simulink model "CryoDetHcd"  (R2016b)
settings: Solver=ode45  StartTime=0.0  StopTime=1e-3  RelTol=1e-3
PreLoadFcn:
  | setup_hcd
values from neighbouring files (symbols this model uses):
  A = sqrt(0.5*erfc(x))    [setup_hcd.m]
  Fadc = 307.2e6    (= 307200000)    [setupADCtoDACloopback.m]    (also in setupCryoFPGA_CMB.m; setup_hcd.m = 614000000)
undefined symbols (not defined in the file or in its folder): AXI4, B, C, D, etaRomData, freqRomData, freqRomData1, freqRomData2, freqRomData3, j, Lite
libraries: xbsIndex_r4 x897, CryoDetLibCMB x8, hdlsllib x8, dspsigops x2, simulink x1
(part 8 of 8)

== system CryoDetHcd/DspCore/DSP/channel_processor/channel_processor_x4/freqWord_debug/alpha_filter1 ==
  In1 : Inport
  alpha : Inport  Port=2
  ch : Inport  Port=3
  (D-A)*B + C : xbsIndex_r4/DSP48 Macro 3.0   dsptype=Target XtremeDSP Slice: DSP48E2  instruction_list=(D-A)*B+C  AvailableInstructions=|  show_filtered=on  pipeline_options=Expert  dspimage=?  tier_1=off  tier_2=off  tier_3=off  tier_4=off  tier_5=off  tier_6=off  dreg_1=off  dreg_2=off  dreg_3=on  areg_1=off  areg_2=off  areg_3=on  areg_4=on  breg_1=off  breg_2=off  breg_3=on  breg_4=on  mreg_5=on  concatreg_3=off  concatreg_4=off  concatreg_5=off  creg_1=off  creg_2=off  creg_3=on  creg_4=on  creg_5=on  preg_6=on  cinreg_1=off  cinreg_2=off  cinreg_3=off  cinreg_4=off  cinreg_5=off  opreg_1=off  opreg_2=off  opreg_3=off  opreg_4=off  opreg_5=off  output_properties=Full_Precision  p_width=48  p_binarywidth=0  has_acout=off  has_bcout=off  has_pcout=off  has_carryout=off  has_carrycascout=off  has_ce=off  has_d_ce=off  has_a_ce=off  has_b_ce=off  has_concat_ce=off  has_c_ce=off  has_m_ce=off  has_p_ce=off  has_sel_ce=off  has_sclr=off  has_d_sclr=off  has_a_sclr=off  has_b_sclr=off  has_concat_sclr=off  has_c_sclr=off  has_m_sclr=off  has_p_sclr=off  has_sel_sclr=off  use_dsp48=on  simulation_type=fast_sim  simulation_model=sysgen:xbip_dsp48_macro_v3_0  gui_behaviour=Sysgen  instruction1='#'  ip_name=DSP48 Macro  ip_version=3.0  dsptool_ready=true  ipcore_usecache=true  ipcore_useipmodelcache=true  wrapper_available=true  port_translation_map={ 'ce' => 'en', 'sclr' => 'rst'}  ipcore_latency_function='has_combinational'  structural_sim=false  ipcore_verbose=false  ipcore_port_config={ 'carryin' => { 'arith' => 'ufix', 'binpt' => 0.00000000000, 'width' => 1.00000000000}, 'carrycascin' => { 'arith' => 'ufix', 'binpt' => 0.00000000000, 'width' => 1.00000000000}, 'carrycascout' => { 'arith' => 'ufix', 'binpt' => 0.00000000000, 'width' => 1.00000000000}, 'carryout' => { 'arith' => 'ufix', 'binpt' => 0.00000000000, 'width' => 1.00000000000}}  ipcore_xco_need_fpga_part=true  block_type=xbip_dsp48_macro_v3_0
      | (D-A)*B+C
      | (D-A)*B+C+C
      | (D-A)*B+C+C+CARRYIN
      | (D-A)*B+C+CARRYIN
      | (D-A)*B+C+P
      | (D-A)*B+C+P+CARRYIN
      | (D-A)*B+C+P>>17
      | (D-A)*B+C+P>>17+CARRYIN
      | (D-A)*B+C+PCIN
      | (D-A)*B+C+PCIN+CARRYIN
      | (D-A)*B+C+PCIN>>17
      | (D-A)*B+C+PCIN>>17+CARRYIN
      | (D-A)*B+C-C
      | (D-A)*B+C-P
      | (D-A)*B+C-P>>17
      | (D-A)*B+C-PCIN
      | (D-A)*B+C-PCIN>>17
      | (D-A)*B+CARRYIN
      | -((D-A)*B+C)
      | -((D-A)*B+C+CARRYIN)
      | -((D-A)*B+CARRYIN)
      | -(C+(D-A)*B+CARRYIN)
      | -(P+(D-A)*B+CARRYIN)
      | -C+(D-A)*B+C
      | -P+(D-A)*B+C
      | -P>>17+(D-A)*B+C
      | -PCIN+(D-A)*B+C
      | -PCIN>>17+(D-A)*B+C
      | C+(D-A)*B+C
      | C+(D-A)*B+C+CARRYIN
      | C+(D-A)*B+CARRYIN
      | C+C+(D-A)*B+CARRYIN
      | C+P+(D-A)*B+CARRYIN
      | C+P>>17+(D-A)*B+CARRYIN
      | C+PCIN+(D-A)*B+CARRYIN
      | C+PCIN>>17+(D-A)*B+CARRYIN
      | C-((D-A)*B+C)
      | C-((D-A)*B+C+CARRYIN)
      | C-((D-A)*B+CARRYIN)
      | C-(C+(D-A)*B+CARRYIN)
      | C-(P+(D-A)*B+CARRYIN)
      | P+(D-A)*B+C
      | P+(D-A)*B+C+CARRYIN
      | P+(D-A)*B+CARRYIN
      | P+C+(D-A)*B+CARRYIN
      | P+P+(D-A)*B+CARRYIN
      | P+P>>17+(D-A)*B+CARRYIN
      | P+PCIN+(D-A)*B+CARRYIN
      | P+PCIN>>17+(D-A)*B+CARRYIN
      | P-((D-A)*B+C)
      | P-((D-A)*B+C+CARRYIN)
      | P-((D-A)*B+CARRYIN)
      | P-(C+(D-A)*B+CARRYIN)
      | P-(P+(D-A)*B+CARRYIN)
      | P>>17+(D-A)*B+C
      | P>>17+(D-A)*B+C+CARRYIN
      | P>>17+(D-A)*B+CARRYIN
      | P>>17+C+(D-A)*B+CARRYIN
      | P>>17+P+(D-A)*B+CARRYIN
      | P>>17-((D-A)*B+C)
      | P>>17-((D-A)*B+C+CARRYIN)
      | P>>17-((D-A)*B+CARRYIN)
      | P>>17-(C+(D-A)*B+CARRYIN)
      | P>>17-(P+(D-A)*B+CARRYIN)
      | PCIN+(D-A)*B+C
      | PCIN+(D-A)*B+C+CARRYIN
      | PCIN+(D-A)*B+CARRYIN
      | PCIN+C+(D-A)*B+CARRYIN
      | PCIN+P+(D-A)*B+CARRYIN
      | PCIN-((D-A)*B+C)
      | PCIN-((D-A)*B+C+CARRYIN)
      | PCIN-((D-A)*B+CARRYIN)
      | PCIN-(C+(D-A)*B+CARRYIN)
      | PCIN-(P+(D-A)*B+CARRYIN)
      | PCIN>>17+(D-A)*B+C
      | PCIN>>17+(D-A)*B+C+CARRYIN
      | PCIN>>17+(D-A)*B+CARRYIN
      | PCIN>>17+C+(D-A)*B+CARRYIN
      | PCIN>>17+P+(D-A)*B+CARRYIN
      | PCIN>>17-((D-A)*B+C)
      | PCIN>>17-((D-A)*B+C+CARRYIN)
      | PCIN>>17-((D-A)*B+CARRYIN)
      | PCIN>>17-(C+(D-A)*B+CARRYIN)
      | PCIN>>17-(P+(D-A)*B+CARRYIN)
      | RNDMACC((D-A)*B+C+P)
      | RNDSIMPLE((D-A)*B+C)
      | RNDSIMPLE((D-A)*B+C+CARRYIN)
      | RNDSIMPLE((D-A)*B+CARRYIN)
      | RNDSIMPLE(C+(D-A)*B+CARRYIN)
      | RNDSIMPLE(P+(D-A)*B+CARRYIN)
      | RNDSIMPLE(P>>17+(D-A)*B+CARRYIN)
      | RNDSIMPLE(PCIN+(D-A)*B+CARRYIN)
      | RNDSIMPLE(PCIN>>17+(D-A)*B+CARRYIN)
      settings: infoedit=<html>Valid operands: CONCAT, P, C, PCIN, P>>17, PCIN>>17, CARRYIN, CARRYCASCIN, ACIN, A, BCIN,B<br><br>Valid operators: +, -, *, ()<br><br>Valid functions: RNDSIMPLE, RNDSYM<br><br>Instructions are case insensitive and tolerate spaces.</html>
  Convert : xbsIndex_r4/Convert  gui_display_data_type=Fixed-point  arith_type=Unsigned  n_bits=24  bin_pt=0  float_type=Single  exp_bits=8  fraction_bits=24  quantization=Truncate  overflow=Wrap  en=off  latency=0  pipeline=off  dbl_ovrd=off  block_type=convert
  Convert1 : xbsIndex_r4/Convert  gui_display_data_type=Fixed-point  arith_type="Signed  (2's comp)"  n_bits=25  bin_pt=0  float_type=Single  exp_bits=8  fraction_bits=24  quantization=Truncate  overflow=Wrap  en=off  latency=0  pipeline=off  dbl_ovrd=off  block_type=convert
  Convert2 : xbsIndex_r4/Convert  gui_display_data_type=Fixed-point  arith_type="Signed  (2's comp)"  n_bits=18  bin_pt=15  float_type=Single  exp_bits=8  fraction_bits=24  quantization=Truncate  overflow=Wrap  en=off  latency=0  pipeline=off  dbl_ovrd=off  block_type=convert
  Convert3 : xbsIndex_r4/Convert  gui_display_data_type=Fixed-point  arith_type="Signed  (2's comp)"  n_bits=25  bin_pt=0  float_type=Single  exp_bits=8  fraction_bits=24  quantization=Truncate  overflow=Wrap  en=off  latency=0  pipeline=off  dbl_ovrd=off  block_type=convert
  Delay : xbsIndex_r4/Delay  rst=off  infoeditControl=Selection of Reset will increase slice count due to use of real FFs and instead of SRLs  en=off  latency=124  reg_retiming=off  dbl_ovrd=off  block_type=delay
  Delay1 : xbsIndex_r4/Delay  rst=off  infoeditControl=Selection of Reset will increase slice count due to use of real FFs and instead of SRLs  en=off  latency=4  reg_retiming=off  dbl_ovrd=off  block_type=delay
  Register : xbsIndex_r4/Register  init=0  rst=off  en=off  dbl_ovrd=off  block_type=register
  Out1 : Outport
  ch_o : Outport  Port=2
  wires:
  alpha/1 -> Convert2/1
  Delay1/1 -> ch_o/1
  ch/1 -> Delay1/1
  Convert3/1 -> (D-A)*B + C/1
  Convert2/1 -> (D-A)*B + C/3
  Convert/1 -> Out1/1
  Convert1/1 -> (D-A)*B + C/2
  (D-A)*B + C/1 -> Delay/1, Convert/1
  Delay/1 -> (D-A)*B + C/4, Convert1/1
  In1/1 -> Register/1
  Register/1 -> Convert3/1

== system CryoDetHcd/DspCore/DSP/channel_processor/channel_processor_x4/freqWord_debug/alpha_filter2 ==
  In1 : Inport
  alpha : Inport  Port=2
  ch : Inport  Port=3
  (D-A)*B + C : xbsIndex_r4/DSP48 Macro 3.0   dsptype=Target XtremeDSP Slice: DSP48E2  instruction_list=(D-A)*B+C  AvailableInstructions=|  show_filtered=on  pipeline_options=Expert  dspimage=?  tier_1=off  tier_2=off  tier_3=off  tier_4=off  tier_5=off  tier_6=off  dreg_1=off  dreg_2=off  dreg_3=on  areg_1=off  areg_2=off  areg_3=on  areg_4=on  breg_1=off  breg_2=off  breg_3=on  breg_4=on  mreg_5=on  concatreg_3=off  concatreg_4=off  concatreg_5=off  creg_1=off  creg_2=off  creg_3=on  creg_4=on  creg_5=on  preg_6=on  cinreg_1=off  cinreg_2=off  cinreg_3=off  cinreg_4=off  cinreg_5=off  opreg_1=off  opreg_2=off  opreg_3=off  opreg_4=off  opreg_5=off  output_properties=Full_Precision  p_width=48  p_binarywidth=0  has_acout=off  has_bcout=off  has_pcout=off  has_carryout=off  has_carrycascout=off  has_ce=off  has_d_ce=off  has_a_ce=off  has_b_ce=off  has_concat_ce=off  has_c_ce=off  has_m_ce=off  has_p_ce=off  has_sel_ce=off  has_sclr=off  has_d_sclr=off  has_a_sclr=off  has_b_sclr=off  has_concat_sclr=off  has_c_sclr=off  has_m_sclr=off  has_p_sclr=off  has_sel_sclr=off  use_dsp48=on  simulation_type=fast_sim  simulation_model=sysgen:xbip_dsp48_macro_v3_0  gui_behaviour=Sysgen  instruction1='#'  ip_name=DSP48 Macro  ip_version=3.0  dsptool_ready=true  ipcore_usecache=true  ipcore_useipmodelcache=true  wrapper_available=true  port_translation_map={ 'ce' => 'en', 'sclr' => 'rst'}  ipcore_latency_function='has_combinational'  structural_sim=false  ipcore_verbose=false  ipcore_port_config={ 'carryin' => { 'arith' => 'ufix', 'binpt' => 0.00000000000, 'width' => 1.00000000000}, 'carrycascin' => { 'arith' => 'ufix', 'binpt' => 0.00000000000, 'width' => 1.00000000000}, 'carrycascout' => { 'arith' => 'ufix', 'binpt' => 0.00000000000, 'width' => 1.00000000000}, 'carryout' => { 'arith' => 'ufix', 'binpt' => 0.00000000000, 'width' => 1.00000000000}}  ipcore_xco_need_fpga_part=true  block_type=xbip_dsp48_macro_v3_0
      | (D-A)*B+C
      | (D-A)*B+C+C
      | (D-A)*B+C+C+CARRYIN
      | (D-A)*B+C+CARRYIN
      | (D-A)*B+C+P
      | (D-A)*B+C+P+CARRYIN
      | (D-A)*B+C+P>>17
      | (D-A)*B+C+P>>17+CARRYIN
      | (D-A)*B+C+PCIN
      | (D-A)*B+C+PCIN+CARRYIN
      | (D-A)*B+C+PCIN>>17
      | (D-A)*B+C+PCIN>>17+CARRYIN
      | (D-A)*B+C-C
      | (D-A)*B+C-P
      | (D-A)*B+C-P>>17
      | (D-A)*B+C-PCIN
      | (D-A)*B+C-PCIN>>17
      | (D-A)*B+CARRYIN
      | -((D-A)*B+C)
      | -((D-A)*B+C+CARRYIN)
      | -((D-A)*B+CARRYIN)
      | -(C+(D-A)*B+CARRYIN)
      | -(P+(D-A)*B+CARRYIN)
      | -C+(D-A)*B+C
      | -P+(D-A)*B+C
      | -P>>17+(D-A)*B+C
      | -PCIN+(D-A)*B+C
      | -PCIN>>17+(D-A)*B+C
      | C+(D-A)*B+C
      | C+(D-A)*B+C+CARRYIN
      | C+(D-A)*B+CARRYIN
      | C+C+(D-A)*B+CARRYIN
      | C+P+(D-A)*B+CARRYIN
      | C+P>>17+(D-A)*B+CARRYIN
      | C+PCIN+(D-A)*B+CARRYIN
      | C+PCIN>>17+(D-A)*B+CARRYIN
      | C-((D-A)*B+C)
      | C-((D-A)*B+C+CARRYIN)
      | C-((D-A)*B+CARRYIN)
      | C-(C+(D-A)*B+CARRYIN)
      | C-(P+(D-A)*B+CARRYIN)
      | P+(D-A)*B+C
      | P+(D-A)*B+C+CARRYIN
      | P+(D-A)*B+CARRYIN
      | P+C+(D-A)*B+CARRYIN
      | P+P+(D-A)*B+CARRYIN
      | P+P>>17+(D-A)*B+CARRYIN
      | P+PCIN+(D-A)*B+CARRYIN
      | P+PCIN>>17+(D-A)*B+CARRYIN
      | P-((D-A)*B+C)
      | P-((D-A)*B+C+CARRYIN)
      | P-((D-A)*B+CARRYIN)
      | P-(C+(D-A)*B+CARRYIN)
      | P-(P+(D-A)*B+CARRYIN)
      | P>>17+(D-A)*B+C
      | P>>17+(D-A)*B+C+CARRYIN
      | P>>17+(D-A)*B+CARRYIN
      | P>>17+C+(D-A)*B+CARRYIN
      | P>>17+P+(D-A)*B+CARRYIN
      | P>>17-((D-A)*B+C)
      | P>>17-((D-A)*B+C+CARRYIN)
      | P>>17-((D-A)*B+CARRYIN)
      | P>>17-(C+(D-A)*B+CARRYIN)
      | P>>17-(P+(D-A)*B+CARRYIN)
      | PCIN+(D-A)*B+C
      | PCIN+(D-A)*B+C+CARRYIN
      | PCIN+(D-A)*B+CARRYIN
      | PCIN+C+(D-A)*B+CARRYIN
      | PCIN+P+(D-A)*B+CARRYIN
      | PCIN-((D-A)*B+C)
      | PCIN-((D-A)*B+C+CARRYIN)
      | PCIN-((D-A)*B+CARRYIN)
      | PCIN-(C+(D-A)*B+CARRYIN)
      | PCIN-(P+(D-A)*B+CARRYIN)
      | PCIN>>17+(D-A)*B+C
      | PCIN>>17+(D-A)*B+C+CARRYIN
      | PCIN>>17+(D-A)*B+CARRYIN
      | PCIN>>17+C+(D-A)*B+CARRYIN
      | PCIN>>17+P+(D-A)*B+CARRYIN
      | PCIN>>17-((D-A)*B+C)
      | PCIN>>17-((D-A)*B+C+CARRYIN)
      | PCIN>>17-((D-A)*B+CARRYIN)
      | PCIN>>17-(C+(D-A)*B+CARRYIN)
      | PCIN>>17-(P+(D-A)*B+CARRYIN)
      | RNDMACC((D-A)*B+C+P)
      | RNDSIMPLE((D-A)*B+C)
      | RNDSIMPLE((D-A)*B+C+CARRYIN)
      | RNDSIMPLE((D-A)*B+CARRYIN)
      | RNDSIMPLE(C+(D-A)*B+CARRYIN)
      | RNDSIMPLE(P+(D-A)*B+CARRYIN)
      | RNDSIMPLE(P>>17+(D-A)*B+CARRYIN)
      | RNDSIMPLE(PCIN+(D-A)*B+CARRYIN)
      | RNDSIMPLE(PCIN>>17+(D-A)*B+CARRYIN)
      settings: infoedit=<html>Valid operands: CONCAT, P, C, PCIN, P>>17, PCIN>>17, CARRYIN, CARRYCASCIN, ACIN, A, BCIN,B<br><br>Valid operators: +, -, *, ()<br><br>Valid functions: RNDSIMPLE, RNDSYM<br><br>Instructions are case insensitive and tolerate spaces.</html>
  Convert : xbsIndex_r4/Convert  gui_display_data_type=Fixed-point  arith_type=Unsigned  n_bits=24  bin_pt=0  float_type=Single  exp_bits=8  fraction_bits=24  quantization=Truncate  overflow=Wrap  en=off  latency=0  pipeline=off  dbl_ovrd=off  block_type=convert
  Convert1 : xbsIndex_r4/Convert  gui_display_data_type=Fixed-point  arith_type="Signed  (2's comp)"  n_bits=25  bin_pt=0  float_type=Single  exp_bits=8  fraction_bits=24  quantization=Truncate  overflow=Wrap  en=off  latency=0  pipeline=off  dbl_ovrd=off  block_type=convert
  Convert2 : xbsIndex_r4/Convert  gui_display_data_type=Fixed-point  arith_type="Signed  (2's comp)"  n_bits=18  bin_pt=15  float_type=Single  exp_bits=8  fraction_bits=24  quantization=Truncate  overflow=Wrap  en=off  latency=0  pipeline=off  dbl_ovrd=off  block_type=convert
  Convert3 : xbsIndex_r4/Convert  gui_display_data_type=Fixed-point  arith_type="Signed  (2's comp)"  n_bits=25  bin_pt=0  float_type=Single  exp_bits=8  fraction_bits=24  quantization=Truncate  overflow=Wrap  en=off  latency=0  pipeline=off  dbl_ovrd=off  block_type=convert
  Delay : xbsIndex_r4/Delay  rst=off  infoeditControl=Selection of Reset will increase slice count due to use of real FFs and instead of SRLs  en=off  latency=124  reg_retiming=off  dbl_ovrd=off  block_type=delay
  Delay1 : xbsIndex_r4/Delay  rst=off  infoeditControl=Selection of Reset will increase slice count due to use of real FFs and instead of SRLs  en=off  latency=4  reg_retiming=off  dbl_ovrd=off  block_type=delay
  Register : xbsIndex_r4/Register  init=0  rst=off  en=off  dbl_ovrd=off  block_type=register
  Out1 : Outport
  ch_o : Outport  Port=2
  wires:
  alpha/1 -> Convert2/1
  Delay1/1 -> ch_o/1
  ch/1 -> Delay1/1
  Convert3/1 -> (D-A)*B + C/1
  Convert2/1 -> (D-A)*B + C/3
  Convert/1 -> Out1/1
  Convert1/1 -> (D-A)*B + C/2
  (D-A)*B + C/1 -> Delay/1, Convert/1
  Delay/1 -> (D-A)*B + C/4, Convert1/1
  In1/1 -> Register/1
  Register/1 -> Convert3/1

== system CryoDetHcd/DspCore/DSP/channel_processor/channel_processor_x4/freqWord_debug/alpha_filter3 ==
  In1 : Inport
  alpha : Inport  Port=2
  ch : Inport  Port=3
  (D-A)*B + C : xbsIndex_r4/DSP48 Macro 3.0   dsptype=Target XtremeDSP Slice: DSP48E2  instruction_list=(D-A)*B+C  AvailableInstructions=|  show_filtered=on  pipeline_options=Expert  dspimage=?  tier_1=off  tier_2=off  tier_3=off  tier_4=off  tier_5=off  tier_6=off  dreg_1=off  dreg_2=off  dreg_3=on  areg_1=off  areg_2=off  areg_3=on  areg_4=on  breg_1=off  breg_2=off  breg_3=on  breg_4=on  mreg_5=on  concatreg_3=off  concatreg_4=off  concatreg_5=off  creg_1=off  creg_2=off  creg_3=on  creg_4=on  creg_5=on  preg_6=on  cinreg_1=off  cinreg_2=off  cinreg_3=off  cinreg_4=off  cinreg_5=off  opreg_1=off  opreg_2=off  opreg_3=off  opreg_4=off  opreg_5=off  output_properties=Full_Precision  p_width=48  p_binarywidth=0  has_acout=off  has_bcout=off  has_pcout=off  has_carryout=off  has_carrycascout=off  has_ce=off  has_d_ce=off  has_a_ce=off  has_b_ce=off  has_concat_ce=off  has_c_ce=off  has_m_ce=off  has_p_ce=off  has_sel_ce=off  has_sclr=off  has_d_sclr=off  has_a_sclr=off  has_b_sclr=off  has_concat_sclr=off  has_c_sclr=off  has_m_sclr=off  has_p_sclr=off  has_sel_sclr=off  use_dsp48=on  simulation_type=fast_sim  simulation_model=sysgen:xbip_dsp48_macro_v3_0  gui_behaviour=Sysgen  instruction1='#'  ip_name=DSP48 Macro  ip_version=3.0  dsptool_ready=true  ipcore_usecache=true  ipcore_useipmodelcache=true  wrapper_available=true  port_translation_map={ 'ce' => 'en', 'sclr' => 'rst'}  ipcore_latency_function='has_combinational'  structural_sim=false  ipcore_verbose=false  ipcore_port_config={ 'carryin' => { 'arith' => 'ufix', 'binpt' => 0.00000000000, 'width' => 1.00000000000}, 'carrycascin' => { 'arith' => 'ufix', 'binpt' => 0.00000000000, 'width' => 1.00000000000}, 'carrycascout' => { 'arith' => 'ufix', 'binpt' => 0.00000000000, 'width' => 1.00000000000}, 'carryout' => { 'arith' => 'ufix', 'binpt' => 0.00000000000, 'width' => 1.00000000000}}  ipcore_xco_need_fpga_part=true  block_type=xbip_dsp48_macro_v3_0
      | (D-A)*B+C
      | (D-A)*B+C+C
      | (D-A)*B+C+C+CARRYIN
      | (D-A)*B+C+CARRYIN
      | (D-A)*B+C+P
      | (D-A)*B+C+P+CARRYIN
      | (D-A)*B+C+P>>17
      | (D-A)*B+C+P>>17+CARRYIN
      | (D-A)*B+C+PCIN
      | (D-A)*B+C+PCIN+CARRYIN
      | (D-A)*B+C+PCIN>>17
      | (D-A)*B+C+PCIN>>17+CARRYIN
      | (D-A)*B+C-C
      | (D-A)*B+C-P
      | (D-A)*B+C-P>>17
      | (D-A)*B+C-PCIN
      | (D-A)*B+C-PCIN>>17
      | (D-A)*B+CARRYIN
      | -((D-A)*B+C)
      | -((D-A)*B+C+CARRYIN)
      | -((D-A)*B+CARRYIN)
      | -(C+(D-A)*B+CARRYIN)
      | -(P+(D-A)*B+CARRYIN)
      | -C+(D-A)*B+C
      | -P+(D-A)*B+C
      | -P>>17+(D-A)*B+C
      | -PCIN+(D-A)*B+C
      | -PCIN>>17+(D-A)*B+C
      | C+(D-A)*B+C
      | C+(D-A)*B+C+CARRYIN
      | C+(D-A)*B+CARRYIN
      | C+C+(D-A)*B+CARRYIN
      | C+P+(D-A)*B+CARRYIN
      | C+P>>17+(D-A)*B+CARRYIN
      | C+PCIN+(D-A)*B+CARRYIN
      | C+PCIN>>17+(D-A)*B+CARRYIN
      | C-((D-A)*B+C)
      | C-((D-A)*B+C+CARRYIN)
      | C-((D-A)*B+CARRYIN)
      | C-(C+(D-A)*B+CARRYIN)
      | C-(P+(D-A)*B+CARRYIN)
      | P+(D-A)*B+C
      | P+(D-A)*B+C+CARRYIN
      | P+(D-A)*B+CARRYIN
      | P+C+(D-A)*B+CARRYIN
      | P+P+(D-A)*B+CARRYIN
      | P+P>>17+(D-A)*B+CARRYIN
      | P+PCIN+(D-A)*B+CARRYIN
      | P+PCIN>>17+(D-A)*B+CARRYIN
      | P-((D-A)*B+C)
      | P-((D-A)*B+C+CARRYIN)
      | P-((D-A)*B+CARRYIN)
      | P-(C+(D-A)*B+CARRYIN)
      | P-(P+(D-A)*B+CARRYIN)
      | P>>17+(D-A)*B+C
      | P>>17+(D-A)*B+C+CARRYIN
      | P>>17+(D-A)*B+CARRYIN
      | P>>17+C+(D-A)*B+CARRYIN
      | P>>17+P+(D-A)*B+CARRYIN
      | P>>17-((D-A)*B+C)
      | P>>17-((D-A)*B+C+CARRYIN)
      | P>>17-((D-A)*B+CARRYIN)
      | P>>17-(C+(D-A)*B+CARRYIN)
      | P>>17-(P+(D-A)*B+CARRYIN)
      | PCIN+(D-A)*B+C
      | PCIN+(D-A)*B+C+CARRYIN
      | PCIN+(D-A)*B+CARRYIN
      | PCIN+C+(D-A)*B+CARRYIN
      | PCIN+P+(D-A)*B+CARRYIN
      | PCIN-((D-A)*B+C)
      | PCIN-((D-A)*B+C+CARRYIN)
      | PCIN-((D-A)*B+CARRYIN)
      | PCIN-(C+(D-A)*B+CARRYIN)
      | PCIN-(P+(D-A)*B+CARRYIN)
      | PCIN>>17+(D-A)*B+C
      | PCIN>>17+(D-A)*B+C+CARRYIN
      | PCIN>>17+(D-A)*B+CARRYIN
      | PCIN>>17+C+(D-A)*B+CARRYIN
      | PCIN>>17+P+(D-A)*B+CARRYIN
      | PCIN>>17-((D-A)*B+C)
      | PCIN>>17-((D-A)*B+C+CARRYIN)
      | PCIN>>17-((D-A)*B+CARRYIN)
      | PCIN>>17-(C+(D-A)*B+CARRYIN)
      | PCIN>>17-(P+(D-A)*B+CARRYIN)
      | RNDMACC((D-A)*B+C+P)
      | RNDSIMPLE((D-A)*B+C)
      | RNDSIMPLE((D-A)*B+C+CARRYIN)
      | RNDSIMPLE((D-A)*B+CARRYIN)
      | RNDSIMPLE(C+(D-A)*B+CARRYIN)
      | RNDSIMPLE(P+(D-A)*B+CARRYIN)
      | RNDSIMPLE(P>>17+(D-A)*B+CARRYIN)
      | RNDSIMPLE(PCIN+(D-A)*B+CARRYIN)
      | RNDSIMPLE(PCIN>>17+(D-A)*B+CARRYIN)
      settings: infoedit=<html>Valid operands: CONCAT, P, C, PCIN, P>>17, PCIN>>17, CARRYIN, CARRYCASCIN, ACIN, A, BCIN,B<br><br>Valid operators: +, -, *, ()<br><br>Valid functions: RNDSIMPLE, RNDSYM<br><br>Instructions are case insensitive and tolerate spaces.</html>
  Convert : xbsIndex_r4/Convert  gui_display_data_type=Fixed-point  arith_type=Unsigned  n_bits=24  bin_pt=0  float_type=Single  exp_bits=8  fraction_bits=24  quantization=Truncate  overflow=Wrap  en=off  latency=0  pipeline=off  dbl_ovrd=off  block_type=convert
  Convert1 : xbsIndex_r4/Convert  gui_display_data_type=Fixed-point  arith_type="Signed  (2's comp)"  n_bits=25  bin_pt=0  float_type=Single  exp_bits=8  fraction_bits=24  quantization=Truncate  overflow=Wrap  en=off  latency=0  pipeline=off  dbl_ovrd=off  block_type=convert
  Convert2 : xbsIndex_r4/Convert  gui_display_data_type=Fixed-point  arith_type="Signed  (2's comp)"  n_bits=18  bin_pt=15  float_type=Single  exp_bits=8  fraction_bits=24  quantization=Truncate  overflow=Wrap  en=off  latency=0  pipeline=off  dbl_ovrd=off  block_type=convert
  Convert3 : xbsIndex_r4/Convert  gui_display_data_type=Fixed-point  arith_type="Signed  (2's comp)"  n_bits=25  bin_pt=0  float_type=Single  exp_bits=8  fraction_bits=24  quantization=Truncate  overflow=Wrap  en=off  latency=0  pipeline=off  dbl_ovrd=off  block_type=convert
  Delay : xbsIndex_r4/Delay  rst=off  infoeditControl=Selection of Reset will increase slice count due to use of real FFs and instead of SRLs  en=off  latency=124  reg_retiming=off  dbl_ovrd=off  block_type=delay
  Delay1 : xbsIndex_r4/Delay  rst=off  infoeditControl=Selection of Reset will increase slice count due to use of real FFs and instead of SRLs  en=off  latency=4  reg_retiming=off  dbl_ovrd=off  block_type=delay
  Register : xbsIndex_r4/Register  init=0  rst=off  en=off  dbl_ovrd=off  block_type=register
  Out1 : Outport
  ch_o : Outport  Port=2
  wires:
  Register/1 -> Convert3/1
  In1/1 -> Register/1
  Delay/1 -> Convert1/1, (D-A)*B + C/4
  (D-A)*B + C/1 -> Convert/1, Delay/1
  Convert1/1 -> (D-A)*B + C/2
  Convert/1 -> Out1/1
  Convert2/1 -> (D-A)*B + C/3
  Convert3/1 -> (D-A)*B + C/1
  ch/1 -> Delay1/1
  Delay1/1 -> ch_o/1
  alpha/1 -> Convert2/1
